simulink model "Modele_SimScape_ControlX"  (R2015a)
settings: Solver=ode15s  StartTime=0.0  StopTime=0.5  RelTol=1e-3
values from neighbouring files (symbols this model uses):
  B = 4    [Modele_SimScape.m]
  Fext = 30    [Modele_SimScape.m]
  Ffrott = 30    [Modele_SimScape.m]
  fv = 20    [Modele_SimScape.m]
  i = 3    [Modele_SimScape.m]
  Jmot = 0.037e-3    (= 3.7e-05)    [Modele_SimScape.m]
  k = 0.21    [Modele_SimScape.m]
  meq = M+Jmot*i^2/R^2    (= 3.19663838502)    [Modele_SimScape.m]
  R = 155/6.28/1000    (= 0.0246815286624)    [Modele_SimScape.m]
undefined symbols (not defined in the file or in its folder): sigbuilder_block
libraries: fl_lib x20, nesl_utility x9, elec_lib x1
settings Model: CovSFcnEnable=off  Creator=Fred  LastModifiedBy=ASUS
settings DebuggingCC: SolverPrmCheckMsg=warning

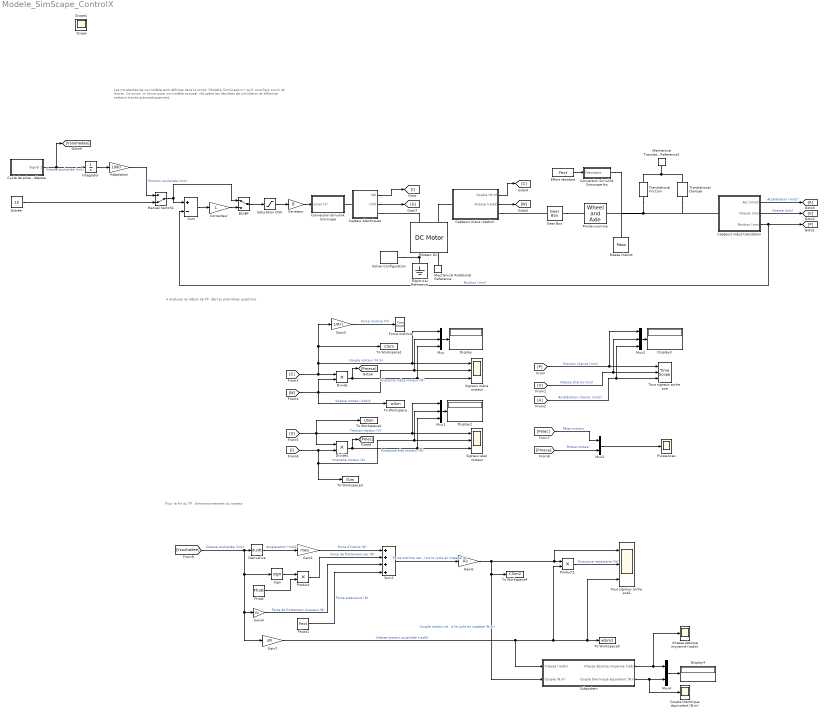
== system Modele_SimScape_ControlX ==
  note: A analyser en début de TP, dès les premières questions
  note: Pour la fin du TP : dimensionnement du moteur
  note: Les constantes de ce modèle sont définies dans le script "Modele_SimScape.m" qu'il vous faut ouvrir et lancer.
      | Ce script .m lance aussi ce modèle acausal, récupère les résultats de simulation et effectue certains tracés automatiquement.
  Adaptation : Gain  Gain=1000
  BO/BF : ManualSwitch
  Capteur électriques : Subsystem
  Capteurs méca rotation : Subsystem
  Capteurs méca translation : Subsystem
  Conversion Simulink Simscape : Subsystem
  Conversion Simulink Simscape bis : Subsystem
  Correcteur : Gain
  Couple thermique équivalent (N.m) : Scope
      settings: ShowLegends=on  TimeRange=1  YMin=-20  YMax=70  SaveName=y4  MaxDataPoints=10001
  Cycle de prise - dépose : Subsystem  Tag=STV Subsys  LoadFcn=sigbuilder_block('load');  StartFcn=sigbuilder_block('start');  StopFcn=sigbuilder_block('stop');  ClipboardFcn=sigbuilder_block('clipboard');  mask(Sigbuilder block){}
      mask help: Simulink:masks:SigbuilderBlock_MD
      mask init:
      | if ~strcmp(get_param(bdroot(gcbh),'SimulationStatus'),'stopped') tuvar = sigbuilder_block('maskInit'); end
      settings: CopyFcn=sigbuilder_block('copy');  DeleteFcn=sigbuilder_block('delete');  ModelCloseFcn=sigbuilder_block('modelClose');  PreSaveFcn=sigbuilder_block('preSave');  PauseFcn=sigbuilder_block('pause');  ContinueFcn=sigbuilder_block('continue');  NameChangeFcn=sigbuilder_block('namechange');  OpenFcn=sigbuilder_block('open',[437.6 199.2 550.4 400 ]);  CloseFcn=sigbuilder_block('close');
      mask Display: plot(0, 0, 100, 100,[2, 2, 32, 32, 2], [68, 8, 8, 68, 68],[32, 2], [38, 38], [32, 19, 2],[53, 60, 44], [32, 17, 17, 2],[16, 16, 31, 31]);txt = getActiveGroup(gcbh);text(2, 100, txt,'verticalAlignment', 'top');
  Derivative : Derivative
  Display{,2..4} (4 alike) : Display
  Divide : Product  Inputs=**
  Divide1 : Product  Inputs=**
  Effort résistant : Constant  Value=Fext
  Electrical Reference : fl_lib/Electrical/Electrical Elements/Electrical Reference
  Entrée : Constant  Value=10
  Ffrott : Constant  Value=Ffrott
  Ffrott1 : Constant  Value=Fext
  "Force motrice " : TimeScope
  Gain1 : Gain  Gain=meq
  Gain3 : Gain  Gain=1/R*i
  Gain4 : Gain  Gain=fv
  Gain6 : Gain  Gain=R/i
  Gain7 : Gain  Gain=i/R
  Gear Box : fl_lib/Mechanical/Mechanisms/Gear Box  ratio=i  t_in_specify=off  t_in_priority=High  t_in=0 N*m  t_out_specify=off  t_out_priority=High  t_out=0 N*m
  Integrator : Integrator
  Manual Switch1 : ManualSwitch  CurrentSetting=0
  Masse chariot : fl_lib/Mechanical/Translational Elements/Mass  mass=M kg  v_specify=on  v_priority=High  v=0 m/s  f_specify=off  f_priority=High  f=0 N
  Mechanical Translational Reference2 : fl_lib/Mechanical/Translational Elements/Mechanical Translational Reference
  Mechanical Rotational Reference : fl_lib/Mechanical/Rotational Elements/Mechanical Rotational Reference
  Moteur DC : elec_lib/Actuators & Drivers/Rotational Actuators/DC Motor  parameterization=1  Ra=r Ohm  La=L H  emf_or_torque=2  Kv=4e-3 V/rpm  Ki=k N*m/A  T_stall=Cmax N*m  w_max=wmax rpm  w_rated=1.5e+4 rpm  P_rated=0.08 W  V_rated=Unom V  J=Jmot kg*m^2  lam_param=1  lam=0 N*m/(rad/s)  i_noload=0 A  V_i_noload=1.5 V  speed0=0 rpm  alpha=0.00393 1/K  Tmeas=25 C  thermal_mass=100 J/K  initial_temperature=25 C
  Mux : Mux  Inputs=3
  Mux1 : Mux  Inputs=3
  Mux2 : Mux  Inputs=2
  Mux3 : Mux  Inputs=3
  Mux4 : Mux  Inputs=2
  Poulie-courroie : fl_lib/Mechanical/Mechanisms/Wheel and Axle  R=R m  or=1  orient=1  t_specify=off  t_priority=High  t=0 N*m  f_specify=off  f_priority=High  f=0 N
  Product : Product
  Product1 : Product
  Puissances : Scope
      settings: ShowLegends=on  YMin=-20  YMax=70  SaveName=y3  MaxDataPoints=10001
  Saturation CNA : Saturate  UpperLimit=10  LowerLimit=-10
  Sign : Signum
  Signaux elec moteur : Scope  NumInputPorts=3
      settings: ShowLegends=on  TimeRange=0.2  YMin=-45~-11~-100  YMax=45~8~450  SaveName=y  MaxDataPoints=10001
  Signaux méca moteur : Scope  NumInputPorts=3
      settings: ShowLegends=on  TimeRange=1  YMin=-20~-5~-5  YMax=70~5~5  SaveName=y6  MaxDataPoints=10001
  Solver Configuration : nesl_utility/Solver Configuration  PhysicalDomain=network_engine_domain  SubClassName=solver  LeftPortType=input  RightPortType=generic  Accelerate=off  Tones=[]  Harmonics=[]  SimulateNoise=off  Profile=off  UseLocalSampling=off  EnableSwitchedLinearOptims=on  FrequencyDomain=off  UseCCode=off  RelTol=0.001  AbsTol=1e-06  MinStep=1e-09  ToWorkspace=off  RevertToSquareIcSolve=off  NumHomotopyIterations=100  DoDC=off  ResidualTolerance=1e-9  UseLocalSolver=off  LocalSolverChoice=NE_BACKWARD_EULER_ADVANCER  LocalSolverSampleTime=.001  DoFixedCost=off  MaxNonlinIter=3  MaxModeIter=2  LinearAlgebra=Sparse  DelaysMemoryBudget=1024  AutomaticFiltering=on  FilteringTimeConstant=0.001
  Subsystem : Subsystem
  Sum : Sum  Inputs=+-
  Sum1 : Sum  Inputs=++++
  To Workspace : ToWorkspace  VariableName=wSim  SampleTime=-1
  To Workspace1 : ToWorkspace  VariableName=CSim  SampleTime=-1
  To Workspace2 : ToWorkspace  VariableName=USim  SampleTime=-1
  To Workspace3 : ToWorkspace  VariableName=ISim  SampleTime=-1
  To Workspace4 : ToWorkspace  VariableName=CSim2  SampleTime=-1
  To Workspace5 : ToWorkspace  VariableName=wSim2  SampleTime=-1
  Tous signaux sortie axe : TimeScope  NumInputPorts=3
  Tous signaux sortie axe1 : Scope  NumInputPorts=3
      settings: ShowLegends=on  TimeRange=1  YMin=-0.85247~-10.9054~-151.935  YMax=0.85247~93.3151~151.935  SaveName=ScopeData2  MaxDataPoints=10001
  Translational Friction : fl_lib/Mechanical/Translational Elements/Translational Friction  brkwy_frc=Ffrott N  Col_frc=Ffrott N  visc_coef=0 N/(m/s)  trans_coef=10 s/m  vel_thr=1e-4 m/s  v_specify=off  v_priority=High  v=0 m/s  f_specify=off  f_priority=High  f=0 N
  Translational Damper : fl_lib/Mechanical/Translational Elements/Translational Damper  D=fv N/(m/s)  v_specify=off  v_priority=High  v=0 m/s  f_specify=off  f_priority=High  f=0 N
  Variateur : Gain  Gain=B
  Vitesse absolue moyenne (rad/s) : Scope
      settings: ShowLegends=on  TimeRange=1  YMin=-20  YMax=70  SaveName=y2  MaxDataPoints=10001
  Scope : Scope
      settings: ShowLegends=on
  Scope1 : Scope
      settings: ShowLegends=on
  wires:
  Divide/1 -> Mux/3, Signaux méca moteur/3, [Pmeca]  "Puissance méca moteur (W)"
  Sum/1 -> Correcteur/1
  Manual Switch1/1 -> BO/BF/1, Sum/1
  Entrée/1 -> Manual Switch1/2
  [V] -> Mux3/2, Tous signaux sortie axe/2  "Vitesse chariot (m/s)"
  [A] -> Mux3/3, Tous signaux sortie axe/3  "Accélération chariot (m/s2)"
  [C] -> Gain3/1, To Workspace1/1, Mux/1, Signaux méca moteur/1, Divide/1  "Couple moteur (N.m)"
  [W] -> Mux/2, Signaux méca moteur/2, To Workspace/1, Divide/2  "Vitesse moteur (rad/s)"
  [Pelec] -> Mux2/1  "Pélec moteur"
  [Pmeca] -> Mux2/2  "Pméca moteur"
  Mux2/1 -> Puissances/1
  Saturation CNA/1 -> Variateur/1
  Gain3/1 -> "Force motrice "/1  "Force motrice (N)"
  Capteurs méca translation/3(Position (mm)) -> Sum/2, [P]  "Position (mm)"
  Capteurs méca translation/1(Acc (m/s2)) -> [A]  "Accélération (m/s2)"
  Capteurs méca rotation/1(Couple (N.m)) -> [C]
  Capteurs méca rotation/2(Vitesse (rad/s)) -> [W]
  Effort résistant/1 -> Conversion Simulink Simscape bis/1(Fresistant)
  Variateur/1 -> Conversion Simulink Simscape/1(Umot (V))
  Capteur électriques/1(I(A)) -> [I]
  Capteur électriques/2(U(V)) -> [U]
  [P] -> Mux3/1, Tous signaux sortie axe/1  "Position chariot (mm)"
  BO/BF/1 -> Saturation CNA/1
  Correcteur/1 -> BO/BF/2
  Integrator/1 -> Adaptation/1
  Cycle de prise - dépose/1(Signal 1) -> Integrator/1, [Vsouhaitee]  "Vitesse souhaitée (m/s)"
  Capteurs méca translation/2(Vitesse (m/s)) -> [V]  "Vitesse (m/s)"
  [Vsouhaitee] -> Gain7/1, Gain4/1, Sign/1, Derivative/1  "Vitesse souhaitée (m/s)"
  Adaptation/1 -> Manual Switch1/1  "Position souhaitée (mm)"
  Derivative/1 -> Gain1/1  "Acceleration (m/s2)"
  Gain1/1 -> Sum1/1  "Force d'inertie (N)"
  Sign/1 -> Product/1
  Product/1 -> Sum1/2  "Force de frottement sec (N)"
  Ffrott/1 -> Product/2
  Gain4/1 -> Sum1/3  "Force de frottement visqueux (N)"
  Ffrott1/1 -> Sum1/4  "Force extérieure (N)"
  Sum1/1 -> Gain6/1  "Force motrice necessaire pour suivre le cycle en trapèze (N)"
  Gain6/1 -> To Workspace4/1, Subsystem/2(Couple (N.m)), Product1/1, Tous signaux sortie axe1/1  "Couple moteur necessaire pour suivre le cycle en trapèze (N.m)"
  Gain7/1 -> Subsystem/1("Vitesse (rad/s) "), Tous signaux sortie axe1/3, To Workspace5/1, Product1/2  "Vitesse moteur souahitée (rad/s)"
  Product1/1 -> Tous signaux sortie axe1/2  "Puissance necessaire (W)"
  Subsystem/1(Vitesse absolue moyenne (rad/s)) -> Mux4/1, Vitesse absolue moyenne (rad/s)/1
  Subsystem/2(Couple thermique équivalent (N.m)) -> Couple thermique équivalent (N.m)/1, Mux4/2
  Mux/1 -> Display/1
  Divide1/1 -> [Pelec], Mux1/3, Signaux elec moteur/3  "Puissance elec moteur (W)"
  [U] -> To Workspace2/1, Divide1/1, Mux1/1, Signaux elec moteur/1  "Tension moteur (V)"
  [I] -> To Workspace3/1, Mux1/2, Signaux elec moteur/2, Divide1/2  "Intensité moteur (A)"
  Mux1/1 -> Display2/1
  Mux3/1 -> Display3/1
  Mux4/1 -> Display4/1
  connections:
  Electrical Reference/LConn1 -- Moteur DC/RConn1 -- Solver Configuration/RConn1
  Gear Box/RConn1 -- Poulie-courroie/LConn1
  Translational Friction/RConn1 -- Translational Damper/LConn1 -- Mechanical Translational Reference2/LConn1
  Translational Friction/LConn1 -- Masse chariot/LConn1 -- Conversion Simulink Simscape bis/RConn1 -- Poulie-courroie/RConn1 -- Capteurs méca translation/LConn1 -- Translational Damper/RConn1
  Capteurs méca rotation/LConn1 -- Moteur DC/LConn2
  Capteurs méca rotation/RConn1 -- Gear Box/LConn1
  Moteur DC/RConn2 -- Mechanical Rotational Reference/LConn1
  Capteur électriques/RConn1 -- Moteur DC/LConn1
  Capteur électriques/LConn1 -- Conversion Simulink Simscape/RConn1

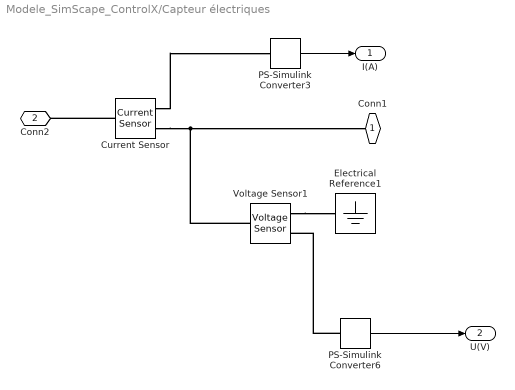
== system Modele_SimScape_ControlX/Capteur électriques ==
  Current Sensor : fl_lib/Electrical/Electrical Sensors/Current Sensor
  Electrical Reference1 : fl_lib/Electrical/Electrical Elements/Electrical Reference
  PS-Simulink Converter3 : nesl_utility/PS-Simulink Converter  PhysicalDomain=network_engine_domain  SubClassName=ps_output  LeftPortType=input  RightPortType=output  PseudoPeriodic=off  Frequencies=[]  Unit=A  AffineConversion=off
  PS-Simulink Converter6 : nesl_utility/PS-Simulink Converter  PhysicalDomain=network_engine_domain  SubClassName=ps_output  LeftPortType=input  RightPortType=output  PseudoPeriodic=off  Frequencies=[]  Unit=1  AffineConversion=off
  Voltage Sensor1 : fl_lib/Electrical/Electrical Sensors/Voltage Sensor
  Conn1 : PMIOPort  Port=1  Side=Right
  Conn2 : PMIOPort  Port=2  Side=Left
  I(A) : Outport
  U(V) : Outport  Port=2
  wires:
  PS-Simulink Converter3/1 -> I(A)/1
  PS-Simulink Converter6/1 -> U(V)/1
  connections:
  Current Sensor/LConn1 -- Conn2/RConn1
  Current Sensor/RConn1 -- PS-Simulink Converter3/LConn1
  Current Sensor/RConn2 -- Conn1/RConn1 -- Voltage Sensor1/LConn1
  PS-Simulink Converter6/LConn1 -- Voltage Sensor1/RConn1
  Voltage Sensor1/RConn2 -- Electrical Reference1/LConn1

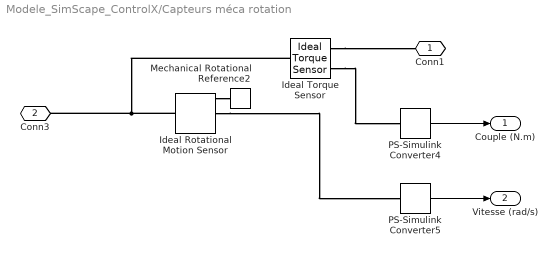
== system Modele_SimScape_ControlX/Capteurs méca rotation ==
  Ideal Rotational Motion Sensor : fl_lib/Mechanical/Mechanical Sensors/Ideal Rotational Motion Sensor  offset=0 rad
  Ideal Torque Sensor : fl_lib/Mechanical/Mechanical Sensors/Ideal Torque Sensor
  Mechanical Rotational Reference2 : fl_lib/Mechanical/Rotational Elements/Mechanical Rotational Reference
  PS-Simulink Converter4 : nesl_utility/PS-Simulink Converter  PhysicalDomain=network_engine_domain  SubClassName=ps_output  LeftPortType=input  RightPortType=output  PseudoPeriodic=off  Frequencies=[]  Unit=N*m  AffineConversion=off
  PS-Simulink Converter5 : nesl_utility/PS-Simulink Converter  PhysicalDomain=network_engine_domain  SubClassName=ps_output  LeftPortType=input  RightPortType=output  PseudoPeriodic=off  Frequencies=[]  Unit=rad/s  AffineConversion=off
  Conn1 : PMIOPort  Port=1  Side=Right
  Conn3 : PMIOPort  Port=2  Side=Left
  Couple (N.m) : Outport
  Vitesse (rad/s) : Outport  Port=2
  wires:
  PS-Simulink Converter4/1 -> Couple (N.m)/1
  PS-Simulink Converter5/1 -> Vitesse (rad/s)/1
  connections:
  Ideal Rotational Motion Sensor/LConn1 -- Ideal Torque Sensor/LConn1 -- Conn3/RConn1
  Ideal Rotational Motion Sensor/RConn2 -- PS-Simulink Converter5/LConn1
  Ideal Torque Sensor/RConn2 -- PS-Simulink Converter4/LConn1
  Ideal Torque Sensor/RConn1 -- Conn1/RConn1
  Ideal Rotational Motion Sensor/RConn1 -- Mechanical Rotational Reference2/LConn1

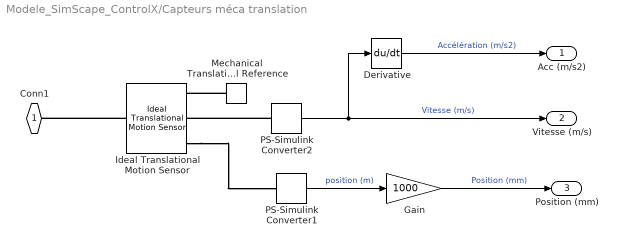
== system Modele_SimScape_ControlX/Capteurs méca translation ==
  Derivative : Derivative
  Gain : Gain  Gain=1000
  Ideal Translational Motion Sensor : fl_lib/Mechanical/Mechanical Sensors/Ideal Translational Motion Sensor  offset=0 m
  Mechanical Translational Reference : fl_lib/Mechanical/Translational Elements/Mechanical Translational Reference
  PS-Simulink Converter1 : nesl_utility/PS-Simulink Converter  PhysicalDomain=network_engine_domain  SubClassName=ps_output  LeftPortType=input  RightPortType=output  PseudoPeriodic=off  Frequencies=[]  Unit=m  AffineConversion=off
  PS-Simulink Converter2 : nesl_utility/PS-Simulink Converter  PhysicalDomain=network_engine_domain  SubClassName=ps_output  LeftPortType=input  RightPortType=output  PseudoPeriodic=off  Frequencies=[]  Unit=m/s  AffineConversion=off
  Conn1 : PMIOPort  Port=1  Side=Left
  Acc (m/s2) : Outport
  Vitesse (m/s) : Outport  Port=2
  Position (mm) : Outport  Port=3
  wires:
  PS-Simulink Converter1/1 -> Gain/1  "position (m)"
  PS-Simulink Converter2/1 -> Vitesse (m/s)/1, Derivative/1  "Vitesse (m/s)"
  Gain/1 -> Position (mm)/1  "Position (mm)"
  Derivative/1 -> Acc (m/s2)/1  "Accélération (m/s2)"
  connections:
  Ideal Translational Motion Sensor/LConn1 -- Conn1/RConn1
  PS-Simulink Converter2/LConn1 -- Ideal Translational Motion Sensor/RConn2
  Ideal Translational Motion Sensor/RConn3 -- PS-Simulink Converter1/LConn1
  Mechanical Translational Reference/LConn1 -- Ideal Translational Motion Sensor/RConn1

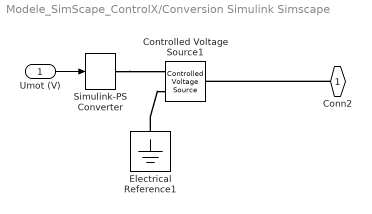
== system Modele_SimScape_ControlX/Conversion Simulink Simscape ==
  Umot (V) : Inport
  Controlled Voltage Source1 : fl_lib/Electrical/Electrical Sources/Controlled Voltage Source
  Electrical Reference1 : fl_lib/Electrical/Electrical Elements/Electrical Reference
  Simulink-PS Converter : nesl_utility/Simulink-PS Converter  PhysicalDomain=network_engine_domain  SubClassName=ps_input  LeftPortType=input  RightPortType=output  PseudoPeriodic=off  Frequencies=[]  NoiseDistribution=none  NoiseParameters=[]  Unit=1  AffineConversion=off  InputFiltering=off  SimscapeFilterOrder=1  InputFilterTimeConstant=0.001  UdotUserProvided=1
  Conn2 : PMIOPort  Port=1  Side=Right
  wires:
  Umot (V)/1 -> Simulink-PS Converter/1
  connections:
  Simulink-PS Converter/RConn1 -- Controlled Voltage Source1/RConn1
  Electrical Reference1/LConn1 -- Controlled Voltage Source1/RConn2
  Conn2/RConn1 -- Controlled Voltage Source1/LConn1

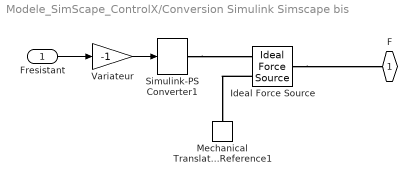
== system Modele_SimScape_ControlX/Conversion Simulink Simscape bis ==
  Fresistant : Inport
  Ideal Force Source : fl_lib/Mechanical/Mechanical Sources/Ideal Force Source
  Mechanical Translational Reference1 : fl_lib/Mechanical/Translational Elements/Mechanical Translational Reference
  Simulink-PS Converter1 : nesl_utility/Simulink-PS Converter  PhysicalDomain=network_engine_domain  SubClassName=ps_input  LeftPortType=input  RightPortType=output  PseudoPeriodic=off  Frequencies=[]  NoiseDistribution=none  NoiseParameters=[]  Unit=N  AffineConversion=off  InputFiltering=off  SimscapeFilterOrder=1  InputFilterTimeConstant=0.001  UdotUserProvided=1
  Variateur : Gain  Gain=-1
  F : PMIOPort  Port=1  Side=Right
  wires:
  Fresistant/1 -> Variateur/1
  Variateur/1 -> Simulink-PS Converter1/1
  connections:
  Ideal Force Source/RConn2 -- Mechanical Translational Reference1/LConn1
  Simulink-PS Converter1/RConn1 -- Ideal Force Source/RConn1
  Ideal Force Source/LConn1 -- F/RConn1

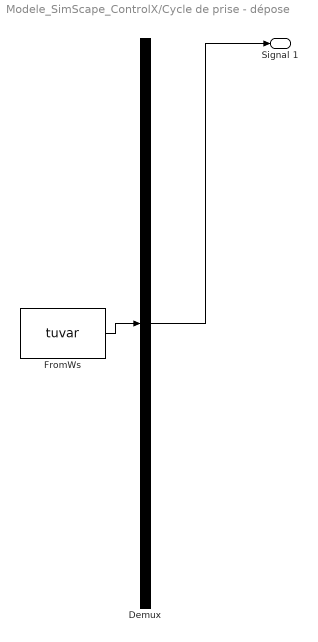
== system Modele_SimScape_ControlX/Cycle de prise - dépose ==
  Demux : Demux  Tag=STV Demux  Outputs=1
  FromWs : FromWorkspace  Tag=STV FromWs  VariableName=tuvar  SampleTime=0
      SigBuilderData=|
      | common.afterFinalStr = 'Extrapolate'
      | common.sampleTime = 0
      | dataSet.timeRange = [0 1]
      | dataSet.name = 'Group 1'
      | sbobj.Groups.Name = 'Group 1'
      | sbobj.Groups.Signals.Name = 'Signal 1'
      | sbobj.Groups.Signals.XData = [0 0.1 0.2 0.4 0.5 0.6 0.7 0.9 1]
      | sbobj.Groups.Signals.YData = [0 0 1 1 0 0 -1 -1 0]
      | sbobj.Groups.TimeRange = [0 1]
  Signal 1 : Outport  Tag=STV Outport
  wires:
  Demux/1 -> Signal 1/1
  FromWs/1 -> Demux/1

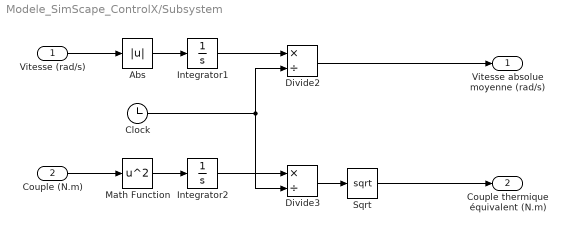
== system Modele_SimScape_ControlX/Subsystem ==
  "Vitesse (rad/s) " : Inport
  Couple (N.m) : Inport  Port=2
  Abs : Abs
  Clock : Clock
  Divide2 : Product  Inputs=*/
  Divide3 : Product  Inputs=*/
  Integrator1 : Integrator
  Integrator2 : Integrator
  Math Function : Math  Operator=square  SaturateOnIntegerOverflow=on
  Sqrt : Sqrt  SaturateOnIntegerOverflow=on
  Vitesse absolue moyenne (rad/s) : Outport
  Couple thermique équivalent (N.m) : Outport  Port=2
  wires:
  Divide3/1 -> Sqrt/1
  Integrator1/1 -> Divide2/1
  Abs/1 -> Integrator1/1
  Math Function/1 -> Integrator2/1
  Integrator2/1 -> Divide3/1
  Couple (N.m)/1 -> Math Function/1
  Divide2/1 -> Vitesse absolue moyenne (rad/s)/1
  "Vitesse (rad/s) "/1 -> Abs/1
  Clock/1 -> Divide3/2, Divide2/2
  Sqrt/1 -> Couple thermique équivalent (N.m)/1
